simulink model "linear_inverted_pendulum_tracking_controller"  (Simulink 7.9)
settings: Solver=ode3  StartTime=0.0  StopTime=8  FixedStep=0.005  RelTol=1e-3
values from neighbouring files (symbols this model uses):
  k1 = -q(1)*q(2)-1    [WPG_results.m]    (also in WPG_results_10.m; WPG_results_2.m; WPG_results_3.m; WPG_results_4.m)
  k2 = (q(1)+q(2))/-q(3)    [WPG_results.m]    (also in WPG_results_10.m; WPG_results_2.m; WPG_results_3.m; WPG_results_4.m)
  k3 = w    [WPG_results.m]    (also in WPG_results_10.m; WPG_results_2.m; WPG_results_3.m; WPG_results_4.m)
  sx_d = [time sx_d]    [WPG_results.m]    (also in WPG_sim.m; control_layer_zmp_com_init.m = [time sx_d_y]; control_layer_zmp_com_init_2.m = [time sx_d_x])
  w = wpg_param.w    [WPG_results.m]    (also in WPG_results_10.m; WPG_results_2.m; WPG_results_3.m; WPG_results_4.m)
  x_d = [time x_d]    [WPG_results.m]    (also in WPG_sim.m; control_layer_zmp_com_init.m = [time x_d_y]; control_layer_zmp_com_init_2.m = [time x_d_x])
libraries: commnoisgen2 x1
settings Model: Creator=pajon  LastModifiedBy=pajon

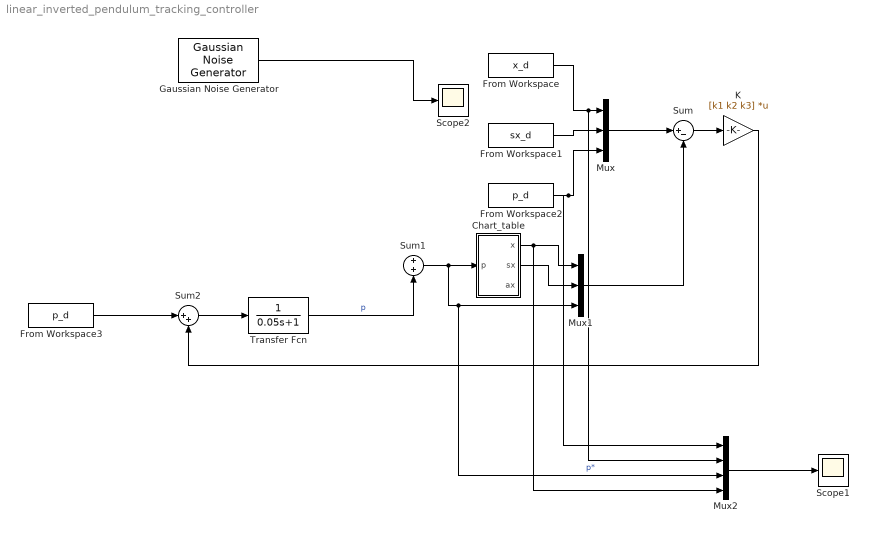
== system linear_inverted_pendulum_tracking_controller ==
  Chart_table : Subsystem
  From Workspace : FromWorkspace  VariableName=x_d  SampleTime=0
  From Workspace1 : FromWorkspace  VariableName=sx_d  SampleTime=0
  From Workspace2 : FromWorkspace  VariableName=p_d  SampleTime=0
  From Workspace3 : FromWorkspace  VariableName=p_d  SampleTime=0
  Gaussian Noise Generator : commnoisgen2/Gaussian Noise Generator  m=0  d=0.001/6  s=41  Ts=0.005  frameBased=off  sampPerFrame=1  orient=off  outDataType=double
  K : Gain  Gain=[k1 k2 k3]  Multiplication=Matrix(K*u)
  Mux : Mux  Inputs=3
  Mux1 : Mux  Inputs=3
  Mux2 : Mux
  Scope1 : Scope
      settings: TimeRange=15
  Scope2 : Scope
      settings: SaveName=ScopeData2
  Sum : Sum  Inputs=|+-
  Sum1 : Sum
  Sum2 : Sum  Inputs=|++
  Transfer Fcn : TransferFcn  Denominator=[0.05 1]
  wires:
  Sum1/1 -> Chart_table/1(p), Mux1/3, Mux2/3  "p*"
  From Workspace/1 -> Mux/1, Mux2/2
  From Workspace1/1 -> Mux/2
  From Workspace2/1 -> Mux/3, Mux2/1
  Mux/1 -> Sum/1
  Mux1/1 -> Sum/2
  Sum/1 -> K/1
  From Workspace3/1 -> Sum2/1
  K/1 -> Sum2/2
  Sum2/1 -> Transfer Fcn/1
  Transfer Fcn/1 -> Sum1/2  "p"
  Chart_table/1(x) -> Mux1/1, Mux2/4
  Chart_table/2(sx) -> Mux1/2
  Mux2/1 -> Scope1/1
  Gaussian Noise Generator/1 -> Scope2/1

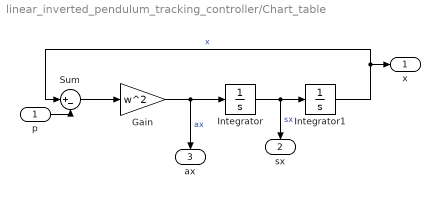
== system linear_inverted_pendulum_tracking_controller/Chart_table ==
  p : Inport
  Gain : Gain  Gain=w^2
  Integrator : Integrator  InitialCondition=sx_d(1,2)
  Integrator1 : Integrator  InitialCondition=x_d(1,2)
  Sum : Sum  Inputs=|+-
  x : Outport
  sx : Outport  Port=2
  ax : Outport  Port=3
  wires:
  Integrator/1 -> Integrator1/1, sx/1  "sx"
  Integrator1/1 -> Sum/1, x/1  "x"
  Gain/1 -> Integrator/1, ax/1  "ax"
  Sum/1 -> Gain/1
  p/1 -> Sum/2
